simulink library "LateralControl_fcns_lib"  (R2018b)
settings: Solver=ode45  StartTime=0.0  StopTime=10.0  RelTol=1e-3  EnableMultiTasking=on
values from neighbouring files (symbols this model uses):
  c_BIT0 = 1.0    [LCK_LogicPara.sldd]
  c_BIT1 = 2.0    [LCK_LogicPara.sldd]
  c_BIT10 = 1024.0    [LCK_LogicPara.sldd]
  c_BIT11 = 2048.0    [LCK_LogicPara.sldd]
  c_BIT12 = 4096.0    [LCK_LogicPara.sldd]
  c_BIT13 = 8192.0    [LCK_LogicPara.sldd]
  c_BIT14 = 16384.0    [LCK_LogicPara.sldd]
  c_BIT15 = 32768.0    [LCK_LogicPara.sldd]
  c_BIT2 = 4.0    [LCK_LogicPara.sldd]
  c_BIT3 = 8.0    [LCK_LogicPara.sldd]
  c_BIT4 = 16.0    [LCK_LogicPara.sldd]
  c_BIT5 = 32.0    [LCK_LogicPara.sldd]
  c_BIT6 = 64.0    [LCK_LogicPara.sldd]
  c_BIT7 = 128.0    [LCK_LogicPara.sldd]
  c_BIT8 = 256.0    [LCK_LogicPara.sldd]
  c_BIT9 = 512.0    [LCK_LogicPara.sldd]
  ML_TIME_MSEC = 20.0    [LCK_Macro.sldd]
undefined symbols (not defined in the file or in its folder): k_LCK_Valid_Range_Remain_Tm_s, k_SPP_clearance_FusGdr, k_SPP_clearance_RE, k_SPP_clearance_VisBarr, TJA_SP_CONF_LOW
libraries: $bdroot x4, simulink x3, tllib x1
(part 1 of 2)
settings Model: TLRevision=101  Creator=kz0hq6  LastModifiedBy=chenx
settings DataIOCC: LimitDataPoints=on  SaveFormat=Array  SignalLoggingSaveFormat=ModelDataLogs
settings OptimizationCC: ExpressionDepthLimit=2147483647  LifeSpan=inf
settings DebuggingCC: UnderspecifiedInitializationDetection=Classic  MergeDetectMultiDrivingBlocksExec=none  SolverPrmCheckMsg=warning  FcnCallInpInsideContextMsg=warning  AllowSymbolicDim=off  StateNameClashWarn=warning  SFUnexpectedBacktrackingDiag=warning  SFNoUnconditionalDefaultTransitionDiag=warning  SFExecutionAtInitializationDiag=none
settings HardwareCC: ProdBitPerPointer=32  ProdBitPerSizeT=32  ProdBitPerPtrDiffT=32  ProdLargestAtomicFloat=None  ProdIntDivRoundTo=Undefined  ProdEndianess=Unspecified  ProdWordSize=32  ProdHWDeviceType=32-bit Generic
settings ModelReferenceCC: PropagateSignalLabelsOutOfModel=off
settings SFSimCC: SimUseLocalCustomCode=off
settings RTWCC: RTWUseLocalCustomCode=off
settings CodeAppCC: StateflowObjectComments=on
settings GRTTargetCC: TargetLangStandard=C89/C90 (ANSI)  GeneratePreprocessorConditionals=Disable all
settings ConfigComp: CovMetricSettings=dw  CovHtmlReporting=on  CovSaveCumulativeToWorkspaceVar=on  CovSaveSingleToWorkspaceVar=on  CovExternalEMLEnable=off

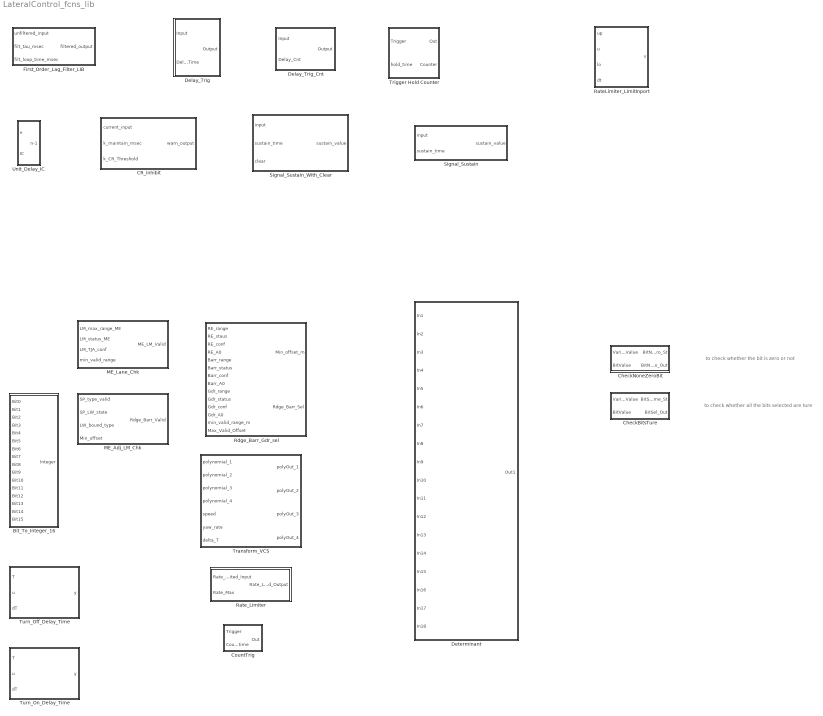
== system LateralControl_fcns_lib ==
  note: to check whether all the bits selected are ture
  note: to check whether the bit is zero or not
  Bit_To_Integer_16 : Subsystem
  CR_inhibit : Subsystem  Description=_GWMAB30P4.Latctrl.000_128_
  CheckBitsTure : Subsystem
  CheckNoneZeroBit : Subsystem
  CountTrig : Subsystem
  Delay_Trig : Subsystem
  Delay_Trig_Cnt : Subsystem  Description=_GWMAB30P4.LKAFN.000_28_
  Determinant : Subsystem
  First_Order_Lag_Filter_LIB : Subsystem
  ME_Adj_LM_Chk : Subsystem
  ME_Lane_Chk : Subsystem
  RateLimiter_LimitInport : Subsystem  mask(Rate Limiter){}
      mask help: Limit rising and falling rates of the signals at the second input by using the first input (upper limit) and the fourth input (lower limit).
      settings: AttributesFormatString=<Rate Limiter>
      mask Display: plot([0.15 0.95],[.5 .5],[.5 .5],[0.05 0.95],0.05+0.9*[.2 .8],0.05+0.9*[0 1]);
  Rate_Limiter : Subsystem  TreatAsAtomicUnit=on
  Rdge_Barr_Gdr_sel : Subsystem
  Signal_Sustain : Subsystem  Description=_GWMAB30P4.LKAFN.000_315_
  Signal_Sustain_With_Clear : Subsystem  Description=_GWMAB30P4.Latctrl.000_162_
  Transform_VCS : Subsystem
  Trigger Hold Counter : Subsystem
  Turn_Off_Delay_Time : Subsystem  mask(TurnOffDelayTime){}
      mask help:
      | The falling edge of the input signal (u) is delayed by the input delay time (T).
      | Input1= Delay Time;  Input2=Signal (u);  Input3=Activation Rate.
      settings: RTWSystemCode=Inline
      mask Help: web(char(which([char(get_param(gcb,'MaskType')),'.html'])));
      mask Display:
      | plot([0.15 0.5 0.5 0.85],[0.9 0.9 0.1 0.1])
      | plot([0.2 0.45],[0.65 0.65])
      | plot([0.325 0.325],[0.65 0.2])
      | port_label('input',1,'T')
      | port_label('input',2,'u')
      | port_label('input',3,'dT')
  Turn_On_Delay_Time : Subsystem  mask(TurnOnDelayTime){}
      mask help: The rising edge of the input signal (u) is delayed by the input delay time (T). Input1= Delay Time; Input2=Signal (u); Input3=Activation Rate.
      settings: RTWSystemCode=Inline
      mask Help: web(char(which([char(get_param(gcb,'MaskType')),'.html'])));
      mask Display:
      | plot([0.15 0.5 0.5 0.85],[0.1 0.1 0.9 0.9])
      | plot([0.55 0.8],[0.65 0.65])
      | plot([0.675 0.675],[0.65 0.2])
      | port_label('input',1,'T')
      | port_label('input',2,'u')
      | port_label('input',3,'dT')
  Unit_Delay_IC : Subsystem

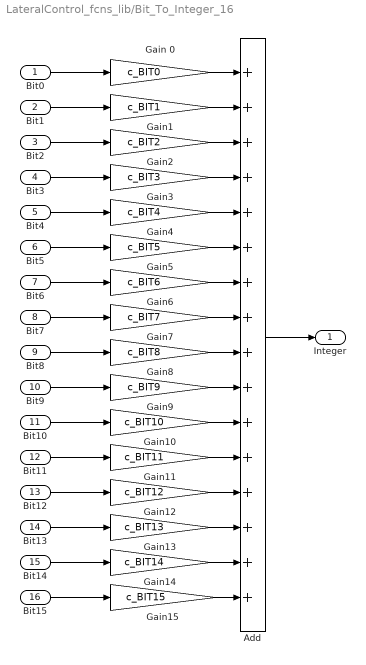
== system LateralControl_fcns_lib/Bit_To_Integer_16 ==
  Bit0 : Inport  Description=_GWMH9P3.LCKFN.000_1_
  Bit1 : Inport  Description=_GWMH9P3.LCKFN.000_2_  Port=2
  Bit2 : Inport  Description=_GWMH9P3.LCKFN.000_3_  Port=3
  Bit3 : Inport  Description=_GWMH9P3.LCKFN.000_4_  Port=4
  Bit4 : Inport  Description=_GWMH9P3.LCKFN.000_5_  Port=5
  Bit5 : Inport  Description=_GWMH9P3.LCKFN.000_6_  Port=6
  Bit6 : Inport  Description=_GWMH9P3.LCKFN.000_7_  Port=7
  Bit7 : Inport  Description=_GWMH9P3.LCKFN.000_8_  Port=8
  Bit8 : Inport  Description=_GWMH9P3.LCKFN.000_9_  Port=9
  Bit9 : Inport  Description=_GWMH9P3.LCKFN.000_10_  Port=10
  Bit10 : Inport  Description=_GWMH9P3.LCKFN.000_11_  Port=11
  Bit11 : Inport  Description=_GWMH9P3.LCKFN.000_12_  Port=12
  Bit12 : Inport  Description=_GWMH9P3.LCKFN.000_13_  Port=13
  Bit13 : Inport  Description=_GWMH9P3.LCKFN.000_14_  Port=14
  Bit14 : Inport  Description=_GWMH9P3.LCKFN.000_15_  Port=15
  Bit15 : Inport  Description=_GWMH9P3.LCKFN.000_16_  Port=16
  Add : Sum  Tag={'output',{'type','UInt16'},'date',737243.50070405088}  Description=_GWMAB30P3.LCKFN.000_1_  Inputs=++++++++++++++++  AccumDataTypeStr=uint16  OutDataTypeStr=uint16
  Gain 0 : Gain  Tag={'output',{'type','UInt16'},'gain',{'name','$P','class','EXTERN_CONST','type','UInt16'},'date',737243.62802085653}  Description=_GWMAB30P3.LCKFN.000_2_  Gain=c_BIT0  ParamDataTypeStr=uint16  OutDataTypeStr=uint16
  Gain1 : Gain  Tag={'output',{'type','UInt16'},'gain',{'name','$P','class','EXTERN_CONST','type','UInt16'},'date',737243.62814724538}  Description=_GWMAB30P3.LCKFN.000_3_  Gain=c_BIT1  ParamDataTypeStr=uint16  OutDataTypeStr=uint16
  Gain10 : Gain  Tag={'output',{'type','UInt16'},'gain',{'name','$P','class','EXTERN_CONST','type','UInt16'},'date',737243.63142819447}  Description=_GWMAB30P3.LCKFN.000_4_  Gain=c_BIT10  ParamDataTypeStr=uint16  OutDataTypeStr=uint16
  Gain11 : Gain  Tag={'output',{'type','UInt16'},'gain',{'name','$P','class','EXTERN_CONST','type','UInt16'},'date',737243.63154284726}  Description=_GWMAB30P3.LCKFN.000_5_  Gain=c_BIT11  ParamDataTypeStr=uint16  OutDataTypeStr=uint16
  Gain12 : Gain  Tag={'output',{'type','UInt16'},'gain',{'name','$P','class','EXTERN_CONST','type','UInt16'},'date',737243.63166906254}  Description=_GWMAB30P3.LCKFN.000_6_  Gain=c_BIT12  ParamDataTypeStr=uint16  OutDataTypeStr=uint16
  Gain13 : Gain  Tag={'output',{'type','UInt16'},'gain',{'name','$P','class','EXTERN_CONST','type','UInt16'},'date',737243.63180953707}  Description=_GWMAB30P3.LCKFN.000_7_  Gain=c_BIT13  ParamDataTypeStr=uint16  OutDataTypeStr=uint16
  Gain14 : Gain  Tag={'output',{'type','UInt16'},'gain',{'name','$P','class','EXTERN_CONST','type','UInt16'},'date',737243.63191913196}  Description=_GWMAB30P3.LCKFN.000_8_  Gain=c_BIT14  ParamDataTypeStr=uint16  OutDataTypeStr=uint16
  Gain15 : Gain  Tag={'output',{'type','UInt16'},'gain',{'name','$P','class','EXTERN_CONST','type','UInt16'},'date',737243.63202458329}  Description=_GWMAB30P3.LCKFN.000_9_  Gain=c_BIT15  ParamDataTypeStr=uint16  OutDataTypeStr=uint16
  Gain2 : Gain  Tag={'output',{'type','UInt16'},'gain',{'name','$P','class','EXTERN_CONST','type','UInt16'},'date',737243.62828194443}  Description=_GWMAB30P3.LCKFN.000_10_  Gain=c_BIT2  ParamDataTypeStr=uint16  OutDataTypeStr=uint16
  Gain3 : Gain  Tag={'output',{'type','UInt16'},'gain',{'name','$P','class','EXTERN_CONST','type','UInt16'},'date',737243.62842260418}  Description=_GWMAB30P3.LCKFN.000_11_  Gain=c_BIT3  ParamDataTypeStr=uint16  OutDataTypeStr=uint16
  Gain4 : Gain  Tag={'output',{'type','UInt16'},'gain',{'name','$P','class','EXTERN_CONST','type','UInt16'},'date',737243.63042121532}  Description=_GWMAB30P3.LCKFN.000_12_  Gain=c_BIT4  ParamDataTypeStr=uint16  OutDataTypeStr=uint16
  Gain5 : Gain  Tag={'output',{'type','UInt16'},'gain',{'name','$P','class','EXTERN_CONST','type','UInt16'},'date',737243.63074442127}  Description=_GWMAB30P3.LCKFN.000_13_  Gain=c_BIT5  ParamDataTypeStr=uint16  OutDataTypeStr=uint16
  Gain6 : Gain  Tag={'output',{'type','UInt16'},'gain',{'name','$P','class','EXTERN_CONST','type','UInt16'},'date',737243.63092443289}  Description=_GWMAB30P3.LCKFN.000_14_  Gain=c_BIT6  ParamDataTypeStr=uint16  OutDataTypeStr=uint16
  Gain7 : Gain  Tag={'output',{'type','UInt16'},'gain',{'name','$P','class','EXTERN_CONST','type','UInt16'},'date',737243.63104162039}  Description=_GWMAB30P3.LCKFN.000_15_  Gain=c_BIT7  ParamDataTypeStr=uint16  OutDataTypeStr=uint16
  Gain8 : Gain  Tag={'output',{'type','UInt16'},'gain',{'name','$P','class','EXTERN_CONST','type','UInt16'},'date',737243.63116565975}  Description=_GWMAB30P3.LCKFN.000_16_  Gain=c_BIT8  ParamDataTypeStr=uint16  OutDataTypeStr=uint16
  Gain9 : Gain  Tag={'output',{'type','UInt16'},'gain',{'name','$P','class','EXTERN_CONST','type','UInt16'},'date',737243.63129422453}  Description=_GWMAB30P3.LCKFN.000_17_  Gain=c_BIT9  ParamDataTypeStr=uint16  OutDataTypeStr=uint16
  Integer : Outport  Description=_GWMH9P3.LCKFN.000_17_
  wires:
  Gain 0/1 -> Add/1
  Gain1/1 -> Add/2
  Gain2/1 -> Add/3
  Gain3/1 -> Add/4
  Gain4/1 -> Add/5
  Gain5/1 -> Add/6
  Gain6/1 -> Add/7
  Gain7/1 -> Add/8
  Gain8/1 -> Add/9
  Gain9/1 -> Add/10
  Gain10/1 -> Add/11
  Gain11/1 -> Add/12
  Gain12/1 -> Add/13
  Gain13/1 -> Add/14
  Gain14/1 -> Add/15
  Gain15/1 -> Add/16
  Add/1 -> Integer/1
  Bit0/1 -> Gain 0/1
  Bit1/1 -> Gain1/1
  Bit2/1 -> Gain2/1
  Bit3/1 -> Gain3/1
  Bit4/1 -> Gain4/1
  Bit5/1 -> Gain5/1
  Bit6/1 -> Gain6/1
  Bit7/1 -> Gain7/1
  Bit8/1 -> Gain8/1
  Bit9/1 -> Gain9/1
  Bit10/1 -> Gain10/1
  Bit11/1 -> Gain11/1
  Bit12/1 -> Gain12/1
  Bit13/1 -> Gain13/1
  Bit14/1 -> Gain14/1
  Bit15/1 -> Gain15/1

== system LateralControl_fcns_lib/CR_inhibit ==
  current_input : Inport  Description=_GWMAB30P4.LKAFN.000_2_
  k_maintain_msec : Inport  Description=_GWMAB30P4.LKAFN.000_3_  Port=2
  k_CR_Threshold : Inport  Description=_GWMAB30P4.LKAFN.000_4_  Port=3
  CR_inhibit : Stateflow chart  Description=_GWMAB30P4.LKAFN.000_5_  TreatAsAtomicUnit=on
  warn_output : Outport  Description=_GWMAB30P4.LKAFN.000_10_
  wires:
  k_CR_Threshold/1 -> CR_inhibit/3(k_CR_Threshold)
  k_maintain_msec/1 -> CR_inhibit/2(k_mantian_msec)
  current_input/1 -> CR_inhibit/1(current_input)
  CR_inhibit/1(warn_output) -> warn_output/1

== system LateralControl_fcns_lib/CheckBitsTure ==
  VariableValue : Inport
  BitValue : Inport  Port=2
  Bitwise Operator5 : simulink/Logic and Bit Operations/Bitwise Operator  logicop=AND  UseBitMask=off  NumInputPorts=2  BitMask=bin2dec('11011001')  BitMaskRealWorld=Stored Integer
  Data Type Conversion26 : DataTypeConversion
  Relational_Operator4 : RelationalOperator  Operator===  OutDataTypeStr=boolean  RndMeth=Nearest
  BitSelSame_St : Outport
  BitSel_Out : Outport  Port=2
  wires:
  BitValue/1 -> Relational_Operator4/2, Data Type Conversion26/1
  VariableValue/1 -> Bitwise Operator5/1
  Relational_Operator4/1 -> BitSelSame_St/1
  Data Type Conversion26/1 -> Bitwise Operator5/2
  Bitwise Operator5/1 -> BitSel_Out/1, Relational_Operator4/1

== system LateralControl_fcns_lib/CheckNoneZeroBit ==
  VariableValue : Inport
  BitValue : Inport  Port=2
  Bitwise AND : simulink/Logic and Bit Operations/Bitwise Operator  logicop=AND  UseBitMask=off  NumInputPorts=2  BitMask=bin2dec('11011001')  BitMaskRealWorld=Stored Integer
  Constant8 : Constant  Value=0
  Data Type Conversion : DataTypeConversion
  Data Type Conversion2 : DataTypeConversion  OutDataTypeStr=uint16
  Relational Operator14 : RelationalOperator  Operator=~=  OutDataTypeStr=boolean  RndMeth=Nearest
  BitNZero_St : Outport
  BitNZero_Out : Outport  Port=2
  wires:
  Data Type Conversion/1 -> Bitwise AND/2
  Relational Operator14/1 -> BitNZero_St/1
  Constant8/1 -> Relational Operator14/2
  BitValue/1 -> Data Type Conversion/1
  Bitwise AND/1 -> Data Type Conversion2/1, Relational Operator14/1
  Data Type Conversion2/1 -> BitNZero_Out/1
  VariableValue/1 -> Bitwise AND/1

== system LateralControl_fcns_lib/CountTrig ==
  Trigger : Inport  Description=_GWMH9P4.LCKFN.000_1_
  Counttrig_time : Inport  Description=_GWMH9P4.LCKFN.000_2_  Port=2
  CountTrig : Stateflow chart  TreatAsAtomicUnit=on
  Out : Outport  Description=_GWMH9P4.LCKFN.000_6_
  wires:
  CountTrig/1(Out) -> Out/1
  Counttrig_time/1 -> CountTrig/2(CountTrig_time)
  Trigger/1 -> CountTrig/1(Trigger)

== system LateralControl_fcns_lib/Delay_Trig ==
  Input : Inport  Description=_GWMH9P3.LCKFN.000_18_
  Delay_Trig_Time : Inport  Description=_GWMH9P3.LCKFN.000_19_  Port=2
  Delay_Trig : Stateflow chart  TreatAsAtomicUnit=on
  Output : Outport  Description=_GWMH9P3.LCKFN.000_23_
  wires:
  Input/1 -> Delay_Trig/1(Input)
  Delay_Trig_Time/1 -> Delay_Trig/2(Delay_Trig_Time)
  Delay_Trig/1(Delay_Trig) -> Output/1

== system LateralControl_fcns_lib/Delay_Trig_Cnt ==
  Input : Inport  Description=_GWMAB30P4.LKAFN.000_29_
  Delay_Cnt : Inport  Description=_GWMAB30P4.LKAFN.000_30_  Port=2
  Delay_Trig : Stateflow chart  Description=_GWMAB30P4.LKAFN.000_31_  TreatAsAtomicUnit=on
  Output : Outport  Description=_GWMAB30P4.LKAFN.000_35_
  wires:
  Delay_Cnt/1 -> Delay_Trig/2(Delay_Trig_count)
  Delay_Trig/1(Delay_Trig) -> Output/1
  Input/1 -> Delay_Trig/1(Input)

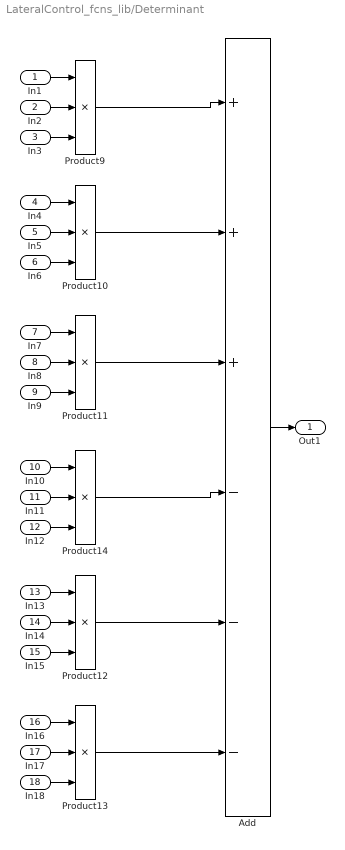
== system LateralControl_fcns_lib/Determinant ==
  In1 : Inport  Tag={'output',{'type','Float32'},'date',737464.8958215625}  Description=_GWMH9P4.LCKFN.000_10_
  In2 : Inport  Tag={'output',{'type','Float32'},'date',737464.8958774074}  Description=_GWMH9P4.LCKFN.000_11_  Port=2
  In3 : Inport  Tag={'output',{'type','Float32'},'date',737464.89607775467}  Description=_GWMH9P4.LCKFN.000_12_  Port=3
  In4 : Inport  Tag={'output',{'type','Float32'},'date',737464.8961349884}  Description=_GWMH9P4.LCKFN.000_13_  Port=4
  In5 : Inport  Tag={'output',{'type','Float32'},'date',737464.89620260417}  Description=_GWMH9P4.LCKFN.000_14_  Port=5
  In6 : Inport  Tag={'output',{'type','Float32'},'date',737464.89625967597}  Description=_GWMH9P4.LCKFN.000_15_  Port=6
  In7 : Inport  Tag={'output',{'type','Float32'},'date',737464.89632886578}  Description=_GWMH9P4.LCKFN.000_16_  Port=7
  In8 : Inport  Tag={'output',{'type','Float32'},'date',737464.89639204857}  Description=_GWMH9P4.LCKFN.000_17_  Port=8
  In9 : Inport  Tag={'output',{'type','Float32'},'date',737464.89645353006}  Description=_GWMH9P4.LCKFN.000_18_  Port=9
  In10 : Inport  Tag={'output',{'type','Float32'},'date',737464.89651208336}  Description=_GWMH9P4.LCKFN.000_19_  Port=10
  In11 : Inport  Tag={'output',{'type','Float32'},'date',737464.89657822915}  Description=_GWMH9P4.LCKFN.000_20_  Port=11
  In12 : Inport  Tag={'output',{'type','Float32'},'date',737464.8966244444}  Description=_GWMH9P4.LCKFN.000_21_  Port=12
  In13 : Inport  Tag={'output',{'type','Float32'},'date',737464.896679456}  Description=_GWMH9P4.LCKFN.000_22_  Port=13
  In14 : Inport  Tag={'output',{'type','Float32'},'date',737464.89673541661}  Description=_GWMH9P4.LCKFN.000_23_  Port=14
  In15 : Inport  Tag={'output',{'type','Float32'},'date',737464.89679289353}  Description=_GWMH9P4.LCKFN.000_24_  Port=15
  In16 : Inport  Tag={'output',{'type','Float32'},'date',737464.89685541671}  Description=_GWMH9P4.LCKFN.000_25_  Port=16
  In17 : Inport  Tag={'output',{'type','Float32'},'date',737464.89690805553}  Description=_GWMH9P4.LCKFN.000_26_  Port=17
  In18 : Inport  Tag={'output',{'type','Float32'},'date',737464.89696628472}  Description=_GWMH9P4.LCKFN.000_27_  Port=18
  Add : Sum  Tag={'output',{'type','Float32'},'date',737462.84083193284}  Description=_GWMH9P4.LCKFN.000_28_  Inputs=+++---
  Product10 : Product  Tag={'output',{'type','Float32'},'date',737462.84057671297}  Description=_GWMH9P4.LCKFN.000_29_  Inputs=3  RndMeth=Zero
  Product11 : Product  Tag={'output',{'type','Float32'},'date',737462.8406229167}  Description=_GWMH9P4.LCKFN.000_30_  Inputs=3  RndMeth=Zero
  Product12 : Product  Tag={'output',{'type','Float32'},'date',737462.84072949074}  Description=_GWMH9P4.LCKFN.000_31_  Inputs=3  RndMeth=Zero
  Product13 : Product  Tag={'output',{'type','Float32'},'date',737462.84078811342}  Description=_GWMH9P4.LCKFN.000_32_  Inputs=3  RndMeth=Zero
  Product14 : Product  Tag={'output',{'type','Float32'},'date',737462.84066295135}  Description=_GWMH9P4.LCKFN.000_33_  Inputs=3  RndMeth=Zero
  Product9 : Product  Tag={'output',{'type','Float32'},'date',737462.8405174769}  Description=_GWMH9P4.LCKFN.000_34_  Inputs=3  RndMeth=Zero
  Out1 : Outport  Tag={'output',{'name','Determinant_out','class','ESR_VC/FCN_RETURN','type','Float32'},'date',737464.89569219912}  Description=_GWMH9P4.LCKFN.000_35_
  wires:
  Product9/1 -> Add/1
  Product10/1 -> Add/2
  Product11/1 -> Add/3
  Product14/1 -> Add/4
  Product12/1 -> Add/5
  Product13/1 -> Add/6
  In1/1 -> Product9/1
  In2/1 -> Product9/2
  In3/1 -> Product9/3
  In4/1 -> Product10/1
  In5/1 -> Product10/2
  In6/1 -> Product10/3
  In7/1 -> Product11/1
  In8/1 -> Product11/2
  In9/1 -> Product11/3
  Add/1 -> Out1/1
  In10/1 -> Product14/1
  In11/1 -> Product14/2
  In12/1 -> Product14/3
  In13/1 -> Product12/1
  In14/1 -> Product12/2
  In15/1 -> Product12/3
  In16/1 -> Product13/1
  In17/1 -> Product13/2
  In18/1 -> Product13/3

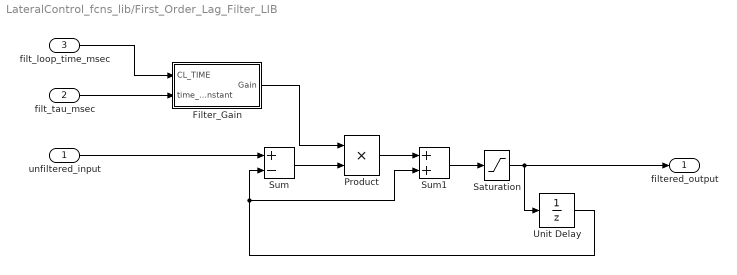
== system LateralControl_fcns_lib/First_Order_Lag_Filter_LIB ==
  unfiltered_input : Inport  Description=_GWMAB30P4.LKAFN.000_148_
  filt_tau_msec : Inport  Description=_GWMAB30P4.LKAFN.000_149_  Port=2
  filt_loop_time_msec : Inport  Description=_GWMAB30P4.LKAFN.000_150_  Port=3
  Filter_Gain : Subsystem
  Product : Product  Description=_GWMAB30P4.LKAFN.000_153_  Inputs=**
  Saturation : Saturate  Description=_GWMAB30P4.LKAFN.000_154_  UpperLimit=65535  LowerLimit=-65535
  Sum : Sum  Description=_GWMAB30P4.LKAFN.000_155_  Inputs=+-  OutDataTypeStr=Inherit: Same as first input
  Sum1 : Sum  Description=_GWMAB30P4.LKAFN.000_156_  OutDataTypeStr=Inherit: Same as first input
  Unit Delay : UnitDelay  Description=_GWMAB30P4.LKAFN.000_157_  SampleTime=-1
  filtered_output : Outport  Description=_GWMAB30P4.LKAFN.000_158_
  wires:
  Filter_Gain/1(Gain) -> Product/1
  Saturation/1 -> filtered_output/1, Unit Delay/1
  Unit Delay/1 -> Sum1/2, Sum/2
  Sum/1 -> Product/2
  Sum1/1 -> Saturation/1
  unfiltered_input/1 -> Sum/1
  filt_tau_msec/1 -> Filter_Gain/2(time_constant)
  Product/1 -> Sum1/1
  filt_loop_time_msec/1 -> Filter_Gain/1(CL_TIME)

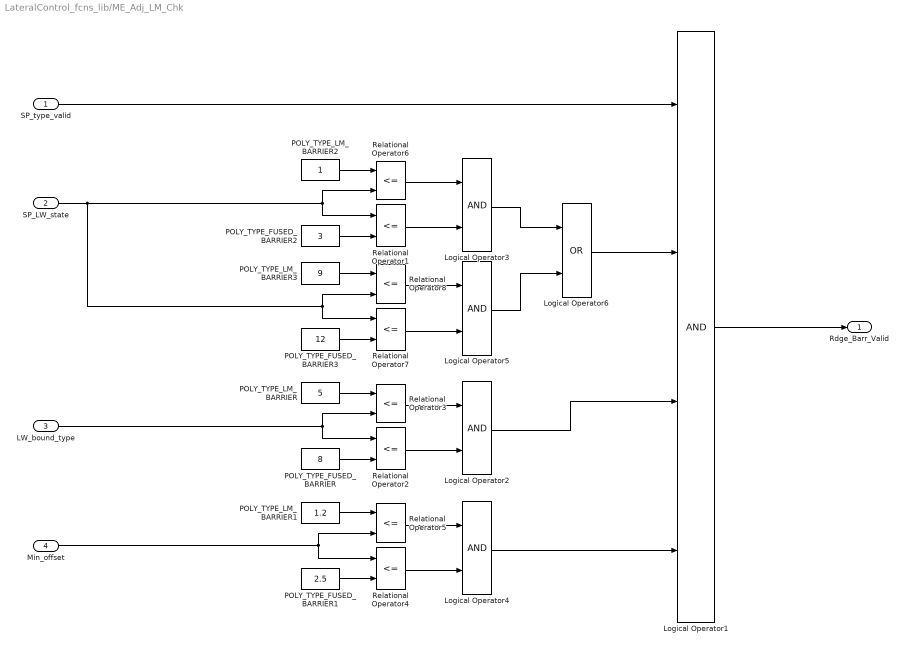
== system LateralControl_fcns_lib/ME_Adj_LM_Chk ==
  SP_type_valid : Inport  Description=_GWMH9P3.LCKFN.000_24_
  SP_LW_state : Inport  Description=_GWMH9P3.LCKFN.000_25_  Port=2
  LW_bound_type : Inport  Description=_GWMH9P3.LCKFN.000_26_  Port=3
  Min_offset : Inport  Description=_GWMH9P3.LCKFN.000_27_  Port=4
  Logical Operator1 : Logic  Tag={'date',737393.51890250004}  Description=_GWMH9P3.LCKFN.000_28_  Inputs=4  AllPortsSameDT=off  OutDataTypeStr=boolean
  Logical Operator2 : Logic  Tag={'date',737393.51890320599}  Description=_GWMH9P3.LCKFN.000_29_  AllPortsSameDT=off  OutDataTypeStr=boolean
  Logical Operator3 : Logic  Tag={'date',737393.51890342589}  Description=_GWMH9P3.LCKFN.000_30_  AllPortsSameDT=off  OutDataTypeStr=boolean
  Logical Operator4 : Logic  Tag={'date',737393.5189036458}  Description=_GWMH9P3.LCKFN.000_31_  AllPortsSameDT=off  OutDataTypeStr=boolean
  Logical Operator5 : Logic  Tag={'date',737393.51890388888}  Description=_GWMH9P3.LCKFN.000_32_  AllPortsSameDT=off  OutDataTypeStr=boolean
  Logical Operator6 : Logic  Tag={'date',737393.51890412043}  Description=_GWMH9P3.LCKFN.000_33_  Operator=OR  AllPortsSameDT=off  OutDataTypeStr=boolean
  POLY_TYPE_FUSED_BARRIER : Constant  Tag={'output',{'type','Int32'},'date',737393.51890491904}  Description=_GWMH9P3.LCKFN.000_34_  Value=8  SampleTime=-1
  POLY_TYPE_FUSED_BARRIER1 : Constant  Tag={'output',{'type','Int32'},'date',737393.51890531252}  Description=_GWMH9P3.LCKFN.000_35_  Value=2.5  SampleTime=-1
  POLY_TYPE_FUSED_BARRIER2 : Constant  Tag={'output',{'type','Int32'},'date',737393.5189055556}  Description=_GWMH9P3.LCKFN.000_36_  Value=3  SampleTime=-1
  POLY_TYPE_FUSED_BARRIER3 : Constant  Tag={'output',{'type','Int32'},'date',737393.51890578703}  Description=_GWMH9P3.LCKFN.000_37_  Value=12  SampleTime=-1
  POLY_TYPE_LM_BARRIER : Constant  Tag={'output',{'type','Int32'},'date',737393.51890601846}  Description=_GWMH9P3.LCKFN.000_38_  Value=5  SampleTime=-1
  POLY_TYPE_LM_BARRIER1 : Constant  Tag={'output',{'type','Int32'},'date',737393.51890626154}  Description=_GWMH9P3.LCKFN.000_39_  Value=1.2  SampleTime=-1
  POLY_TYPE_LM_BARRIER2 : Constant  Tag={'output',{'type','Int32'},'date',737393.51890650461}  Description=_GWMH9P3.LCKFN.000_40_  SampleTime=-1
  POLY_TYPE_LM_BARRIER3 : Constant  Tag={'output',{'type','Int32'},'date',737393.51890672452}  Description=_GWMH9P3.LCKFN.000_41_  Value=9  SampleTime=-1
  Relational Operator1 : RelationalOperator  Tag={'date',737393.51890695607}  Description=_GWMH9P3.LCKFN.000_42_  Operator=<=  OutDataTypeStr=boolean  RndMeth=Nearest
  Relational Operator2 : RelationalOperator  Tag={'date',737393.51890716434}  Description=_GWMH9P3.LCKFN.000_43_  Operator=<=  OutDataTypeStr=boolean  RndMeth=Nearest
  Relational Operator3 : RelationalOperator  Tag={'date',737393.51890737272}  Description=_GWMH9P3.LCKFN.000_44_  Operator=<=  OutDataTypeStr=boolean  RndMeth=Nearest
  Relational Operator4 : RelationalOperator  Tag={'date',737393.51890755782}  Description=_GWMH9P3.LCKFN.000_45_  Operator=<=  OutDataTypeStr=boolean  RndMeth=Nearest
  Relational Operator5 : RelationalOperator  Tag={'date',737393.51890776621}  Description=_GWMH9P3.LCKFN.000_46_  Operator=<=  OutDataTypeStr=boolean  RndMeth=Nearest
  Relational Operator6 : RelationalOperator  Tag={'date',737393.51890796295}  Description=_GWMH9P3.LCKFN.000_47_  Operator=<=  OutDataTypeStr=boolean  RndMeth=Nearest
  Relational Operator7 : RelationalOperator  Tag={'date',737393.51890815969}  Description=_GWMH9P3.LCKFN.000_48_  Operator=<=  OutDataTypeStr=boolean  RndMeth=Nearest
  Relational Operator8 : RelationalOperator  Tag={'date',737393.51890836807}  Description=_GWMH9P3.LCKFN.000_49_  Operator=<=  OutDataTypeStr=boolean  RndMeth=Nearest
  Rdge_Barr_Valid : Outport  Description=_GWMH9P3.LCKFN.000_50_
  wires:
  Logical Operator1/1 -> Rdge_Barr_Valid/1
  LW_bound_type/1 -> Relational Operator2/1, Relational Operator3/2
  POLY_TYPE_FUSED_BARRIER/1 -> Relational Operator2/2
  POLY_TYPE_LM_BARRIER/1 -> Relational Operator3/1
  Relational Operator2/1 -> Logical Operator2/2
  Relational Operator3/1 -> Logical Operator2/1
  Min_offset/1 -> Relational Operator5/2, Relational Operator4/1
  POLY_TYPE_FUSED_BARRIER1/1 -> Relational Operator4/2
  POLY_TYPE_LM_BARRIER1/1 -> Relational Operator5/1
  Relational Operator4/1 -> Logical Operator4/2
  Relational Operator5/1 -> Logical Operator4/1
  SP_LW_state/1 -> Relational Operator6/2, Relational Operator1/1, Relational Operator7/1, Relational Operator8/2
  POLY_TYPE_FUSED_BARRIER2/1 -> Relational Operator1/2
  POLY_TYPE_LM_BARRIER2/1 -> Relational Operator6/1
  Relational Operator1/1 -> Logical Operator3/2
  Relational Operator6/1 -> Logical Operator3/1
  POLY_TYPE_FUSED_BARRIER3/1 -> Relational Operator7/2
  POLY_TYPE_LM_BARRIER3/1 -> Relational Operator8/1
  Relational Operator7/1 -> Logical Operator5/2
  Relational Operator8/1 -> Logical Operator5/1
  Logical Operator3/1 -> Logical Operator6/1
  Logical Operator5/1 -> Logical Operator6/2
  SP_type_valid/1 -> Logical Operator1/1
  Logical Operator6/1 -> Logical Operator1/2
  Logical Operator2/1 -> Logical Operator1/3
  Logical Operator4/1 -> Logical Operator1/4

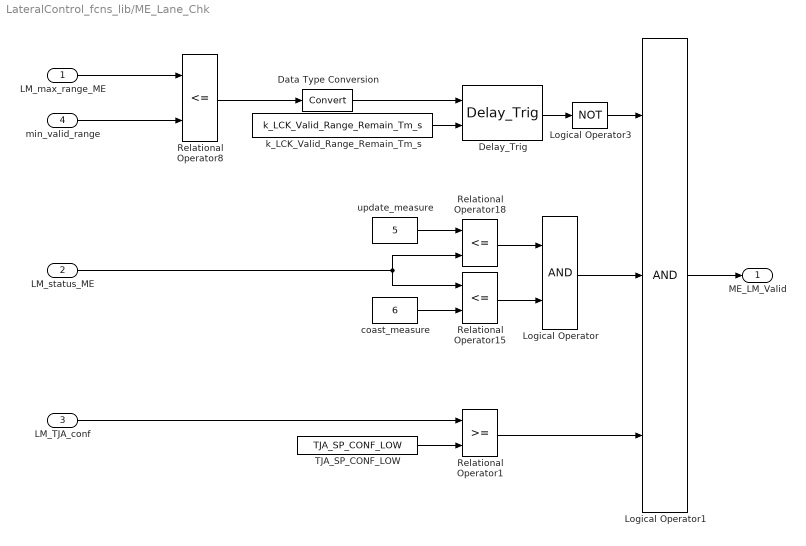
== system LateralControl_fcns_lib/ME_Lane_Chk ==
  LM_max_range_ME : Inport  Tag={'output',{'name','$I_LM_max_range_ME','type','Float32'},'date',737429.7295920949}  Description=_GWMH9P3.LCKFN.000_51_
  LM_status_ME : Inport  Tag={'output',{'name','$I_LM_status_ME','type','UInt8'},'date',737429.72993736109}  Description=_GWMH9P3.LCKFN.000_52_  Port=2
  LM_TJA_conf : Inport  Tag={'output',{'name','$I_LM_TJA_conf','type','UInt8'},'date',737429.73083754629}  Description=_GWMH9P3.LCKFN.000_53_  Port=3
  min_valid_range : Inport  Tag={'output',{'name','$I_min_valid_range','type','UInt8'},'date',737429.72976344905}  Description=_GWMH9P3.LCKFN.000_54_  Port=4
  Data Type Conversion : DataTypeConversion  Description=_GWMH9P3.LCKFN.000_55_
  Delay_Trig : $bdroot/Delay_Trig  SystemSampleTime=-1
  Logical Operator : Logic  Tag={'date',737237.63446607639}  Description=_GWMAB30P3.LCKFN.000_18_  AllPortsSameDT=off  OutDataTypeStr=boolean
  Logical Operator1 : Logic  Tag={'date',737237.63446620374}  Description=_GWMAB30P3.LCKFN.000_19_  Inputs=3  AllPortsSameDT=off  OutDataTypeStr=boolean
  Logical Operator3 : Logic  Tag={'date',737237.63446633099}  Description=_GWMAB30P3.LCKFN.000_20_  Operator=NOT  Inputs=1  AllPortsSameDT=off  OutDataTypeStr=boolean
  Relational Operator1 : RelationalOperator  Tag={'date',737237.6344665857}  Description=_GWMAB30P3.LCKFN.000_21_  OutDataTypeStr=boolean  RndMeth=Nearest
  Relational Operator15 : RelationalOperator  Tag={'date',737237.63446671295}  Description=_GWMAB30P3.LCKFN.000_22_  Operator=<=  OutDataTypeStr=boolean  RndMeth=Nearest
  Relational Operator18 : RelationalOperator  Tag={'date',737237.63446682866}  Description=_GWMAB30P3.LCKFN.000_23_  Operator=<=  OutDataTypeStr=boolean  RndMeth=Nearest
  Relational Operator8 : RelationalOperator  Tag={'date',737237.63446693285}  Description=_GWMAB30P3.LCKFN.000_24_  Operator=<=  OutDataTypeStr=boolean  RndMeth=Nearest
  TJA_SP_CONF_LOW : Constant  Tag={'output',{'name','$P','class','EXTERN_MACRO','type','UInt8'},'date',737237.8042558796}  Description=_GWMAB30P3.LCKFN.000_25_  Value=TJA_SP_CONF_LOW  SampleTime=-1
  coast_measure : Constant  Tag={'output',{'type','Int32'},'date',737237.6344671991}  Description=_GWMAB30P3.LCKFN.000_26_  Value=6  SampleTime=-1
  k_LCK_Valid_Range_Remain_Tm_s : Constant  Tag={'output',{'name','$P','class','EXTERN_CAL','type','Float32'},'date',737237.80413560185}  Description=_GWMAB30P3.LCKFN.000_27_  Value=k_LCK_Valid_Range_Remain_Tm_s  SampleTime=-1
  update_measure : Constant  Tag={'output',{'type','Int32'},'date',737237.63446748839}  Description=_GWMAB30P3.LCKFN.000_28_  Value=5  SampleTime=-1
  ME_LM_Valid : Outport  Tag={'output',{'name','$I_ME_LM_Valid','class','ESR_VC/FCN_RETURN','type','Bool'},'date',737429.72934129625}  Description=_GWMH9P3.LCKFN.000_56_
  wires:
  min_valid_range/1 -> Relational Operator8/2
  LM_max_range_ME/1 -> Relational Operator8/1
  LM_status_ME/1 -> Relational Operator18/2, Relational Operator15/1
  coast_measure/1 -> Relational Operator15/2
  update_measure/1 -> Relational Operator18/1
  LM_TJA_conf/1 -> Relational Operator1/1
  TJA_SP_CONF_LOW/1 -> Relational Operator1/2
  Relational Operator15/1 -> Logical Operator/2
  Relational Operator18/1 -> Logical Operator/1
  Logical Operator/1 -> Logical Operator1/2
  Relational Operator1/1 -> Logical Operator1/3
  Logical Operator1/1 -> ME_LM_Valid/1
  Relational Operator8/1 -> Data Type Conversion/1
  Logical Operator3/1 -> Logical Operator1/1
  Delay_Trig/1 -> Logical Operator3/1
  k_LCK_Valid_Range_Remain_Tm_s/1 -> Delay_Trig/2
  Data Type Conversion/1 -> Delay_Trig/1

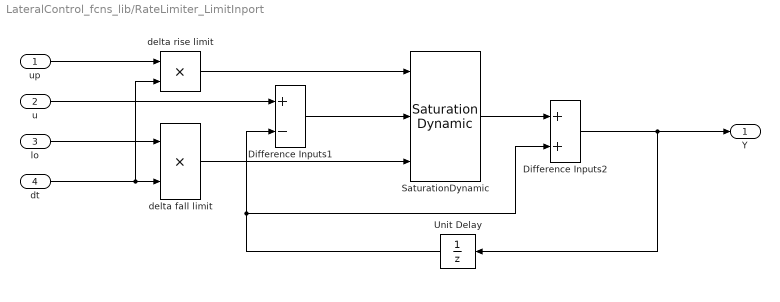
== system LateralControl_fcns_lib/RateLimiter_LimitInport ==
  up : Inport
  u : Inport  Port=2
  lo : Inport  Port=3
  dt : Inport  Port=4
  Difference Inputs1 : Sum  Description=Add in CPU  Inputs=+-  OutDataTypeStr=Inherit: Inherit via back propagation  RndMeth=Zero
  Difference Inputs2 : Sum  Description=Add in CPU  OutDataTypeStr=Inherit: Inherit via back propagation  RndMeth=Zero
  SaturationDynamic : simulink/Discontinuities/Saturation Dynamic  OutMin=[]  OutMax=[]  OutDataTypeStr=Inherit: Same as second input  OutDataType=fixdt(1, 16)  OutScaling=2^-10  RndMeth=Zero  DoSatur=off
  Unit Delay : UnitDelay  SampleTime=-1
  delta fall limit : Product  Inputs=**  OutDataTypeStr=Inherit: Inherit via back propagation  SaturateOnIntegerOverflow=on  RndMeth=Zero
  delta rise limit : Product  Inputs=**  OutDataTypeStr=Inherit: Inherit via back propagation  SaturateOnIntegerOverflow=on  RndMeth=Zero
  Y : Outport  InitialOutput=0
  wires:
  Difference Inputs1/1 -> SaturationDynamic/2
  u/1 -> Difference Inputs1/1
  delta fall limit/1 -> SaturationDynamic/3
  SaturationDynamic/1 -> Difference Inputs2/1
  Unit Delay/1 -> Difference Inputs1/2, Difference Inputs2/2
  Difference Inputs2/1 -> Unit Delay/1, Y/1
  up/1 -> delta rise limit/1
  delta rise limit/1 -> SaturationDynamic/1
  lo/1 -> delta fall limit/1
  dt/1 -> delta fall limit/2, delta rise limit/2

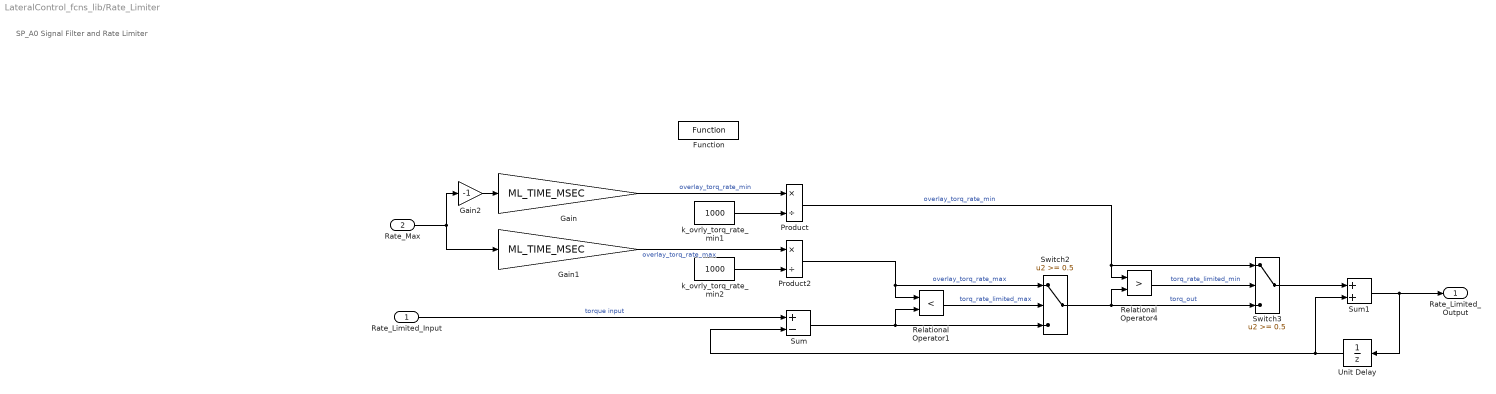
== system LateralControl_fcns_lib/Rate_Limiter ==
  note: SP_A0 Signal Filter and Rate Limiter
  Rate_Limited_Input : Inport  Description=_GWMH9P4.LCKFN.000_36_
  Rate_Max : Inport  Description=_GWMH9P4.LCKFN.000_37_  Port=2
  Function : tllib/Function
  Gain : Gain  Tag={'output',{'type','Float32'},'gain',{'name','$P','class','EXTERN_MACRO','type','ESR_Typedefs/unsigned8_T'},'date',737464.50571820606}  Description=_GWMH9P4.LCKFN.000_38_  Gain=ML_TIME_MSEC
  Gain1 : Gain  Tag={'output',{'type','Float32'},'gain',{'name','$P','class','EXTERN_MACRO','type','ESR_Typedefs/unsigned8_T'},'date',737464.50596844906}  Description=_GWMH9P4.LCKFN.000_39_  Gain=ML_TIME_MSEC
  Gain2 : Gain  Tag={'output',{'type','Float32'},'gain',{'type','Int32'},'date',737462.83431409718}  Description=_GWMH9P4.LCKFN.000_40_  Gain=-1
  Product : Product  Tag={'output',{'type','Float32'},'exceptionhandling',0,'date',737462.83562771988}  Description=_GWMH9P4.LCKFN.000_41_  Inputs=*/  InputSameDT=on  OutDataTypeStr=Inherit: Same as first input
  Product2 : Product  Tag={'output',{'type','Float32'},'exceptionhandling',0,'date',737462.83566040511}  Description=_GWMH9P4.LCKFN.000_42_  Inputs=*/  InputSameDT=on  OutDataTypeStr=Inherit: Same as first input
  Relational Operator1 : RelationalOperator  Tag={'date',737462.49266613426}  Description=_GWMH9P4.LCKFN.000_43_  Operator=<  RndMeth=Nearest
  Relational Operator4 : RelationalOperator  Tag={'date',737462.49266649305}  Description=_GWMH9P4.LCKFN.000_44_  Operator=>  RndMeth=Nearest
  Sum : Sum  Tag={'output',{'type','Float32'},'date',737462.83688239579}  Description=_GWMH9P4.LCKFN.000_45_  Inputs=+-  InputSameDT=on  OutDataTypeStr=Inherit: Same as first input
  Sum1 : Sum  Tag={'output',{'type','Float32'},'date',737462.83708119218}  Description=_GWMH9P4.LCKFN.000_46_  InputSameDT=on  OutDataTypeStr=Inherit: Same as first input
  Switch2 : Switch  Tag={'output',{'type','Float32'},'threshold',{'type','Int32'},'date',737462.8369607986}  Description=_GWMH9P4.LCKFN.000_47_  Threshold=0.5  OutDataTypeStr=Inherit: Inherit via back propagation
  Switch3 : Switch  Tag={'output',{'type','Float32'},'threshold',{'type','Int32'},'date',737462.83703094907}  Description=_GWMH9P4.LCKFN.000_48_  Threshold=0.5  OutDataTypeStr=Inherit: Inherit via back propagation
  Unit Delay : UnitDelay  Tag={'output',{'inheritscaling',1},'date',737462.6251862963}  Description=_GWMH9P4.LCKFN.000_49_  SampleTime=-1
  k_ovrly_torq_rate_min1 : Constant  Tag={'output',{'type','Int32'},'date',737462.8361334838}  Description=_GWMH9P4.LCKFN.000_50_  Value=1000
  k_ovrly_torq_rate_min2 : Constant  Tag={'output',{'type','Int32'},'date',737462.8361574884}  Description=_GWMH9P4.LCKFN.000_51_  Value=1000
  Rate_Limited_Output : Outport  Description=_GWMH9P4.LCKFN.000_52_
  wires:
  k_ovrly_torq_rate_min2/1 -> Product2/2
  Gain1/1 -> Product2/1  "overlay_torq_rate_max"
  k_ovrly_torq_rate_min1/1 -> Product/2
  Gain/1 -> Product/1  "overlay_torq_rate_min"
  Relational Operator1/1 -> Switch2/2  "torq_rate_limited_max"
  Switch2/1 -> Relational Operator4/2, Switch3/3  "torq_out"
  Relational Operator4/1 -> Switch3/2  "torq_rate_limited_min"
  Gain2/1 -> Gain/1
  Product2/1 -> Relational Operator1/1, Switch2/1  "overlay_torq_rate_max"
  Product/1 -> Relational Operator4/1, Switch3/1  "overlay_torq_rate_min"
  Switch3/1 -> Sum1/1
  Sum/1 -> Relational Operator1/2, Switch2/3
  Unit Delay/1 -> Sum/2, Sum1/2
  Sum1/1 -> Rate_Limited_Output/1, Unit Delay/1
  Rate_Limited_Input/1 -> Sum/1  "torque input"
  Rate_Max/1 -> Gain2/1, Gain1/1

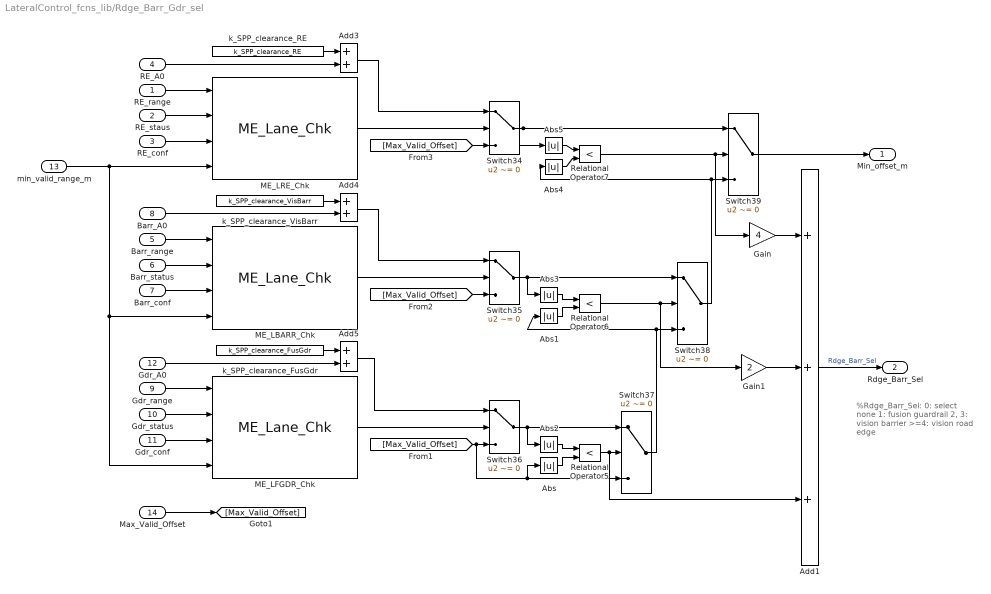
== system LateralControl_fcns_lib/Rdge_Barr_Gdr_sel ==
  note: %Rdge_Barr_Sel:
      | 0:       select none
      | 1:       fusion guardrail
      | 2, 3:   vision barrier
      | >=4:   vision road edge
  RE_range : Inport  Tag={'output',{'name','$I_RE_range','class','ESR_VC/FCN_ARG','type','Float32'},'date',737395.78900525463}  Description=_GWMH9P3.LCKFN.000_57_
  RE_staus : Inport  Tag={'output',{'name','$I_RE_Status','class','ESR_VC/FCN_ARG','type','UInt8'},'date',737395.7890536458}  Description=_GWMH9P3.LCKFN.000_58_  Port=2
  RE_conf : Inport  Tag={'output',{'name','$I_RE_conf','class','ESR_VC/FCN_ARG','type','UInt8'},'date',737395.78910004627}  Description=_GWMH9P3.LCKFN.000_59_  Port=3
  RE_A0 : Inport  Tag={'output',{'name','$I_RE_A0','class','ESR_VC/FCN_ARG','type','Float32'},'date',737395.78706298606}  Description=_GWMH9P3.LCKFN.000_60_  Port=4
  Barr_range : Inport  Tag={'output',{'name','$I_Barr_range','class','ESR_VC/FCN_ARG','type','Float32'},'date',737395.79003777774}  Description=_GWMH9P3.LCKFN.000_61_  Port=5
  Barr_status : Inport  Tag={'output',{'name','$I_Barr_status','class','ESR_VC/FCN_ARG','type','UInt8'},'date',737395.79025012732}  Description=_GWMH9P3.LCKFN.000_62_  Port=6
  Barr_conf : Inport  Tag={'output',{'name','$I_Barr_conf','class','ESR_VC/FCN_ARG','type','UInt8'},'date',737395.79030952544}  Description=_GWMH9P3.LCKFN.000_63_  Port=7
  Barr_A0 : Inport  Tag={'output',{'name','$I_Barr_A0','class','ESR_VC/FCN_ARG','type','Float32'},'date',737395.79016039358}  Description=_GWMH9P3.LCKFN.000_64_  Port=8
  Gdr_range : Inport  Tag={'output',{'name','$I_Gdr_range','type','Float32'},'date',737395.79107519682}  Description=_GWMH9P3.LCKFN.000_65_  Port=9
  Gdr_status : Inport  Tag={'output',{'name','$I_Gdr_status','class','ESR_VC/FCN_ARG','type','UInt8'},'date',737395.79137348384}  Description=_GWMH9P3.LCKFN.000_66_  Port=10
  Gdr_conf : Inport  Tag={'output',{'name','$I_Gdr_conf','class','ESR_VC/FCN_ARG','type','UInt8'},'date',737395.7916990394}  Description=_GWMH9P3.LCKFN.000_67_  Port=11
  Gdr_A0 : Inport  Tag={'output',{'name','$I_Gdr_A0','class','ESR_VC/FCN_ARG','type','Float32'},'date',737395.7909677662}  Description=_GWMH9P3.LCKFN.000_68_  Port=12
  min_valid_range_m : Inport  Tag={'output',{'name','$I_min_valid_range_m','class','ESR_VC/FCN_ARG','type','UInt8'},'date',737395.78932809026}  Description=_GWMH9P3.LCKFN.000_69_  Port=13
  Max_Valid_Offset : Inport  Tag={'output',{'name','$I_Max_Valid_Offset','class','ESR_VC/FCN_ARG'},'date',737395.79202499997}  Description=_GWMH9P3.LCKFN.000_70_  Port=14
  Abs : Abs  Tag={'output',{'type','Float32'},'date',737394.50935303245}  Description=_GWMH9P3.LCKFN.000_71_
  Abs1 : Abs  Tag={'output',{'type','Float32'},'date',737394.50935375004}  Description=_GWMH9P3.LCKFN.000_72_
  Abs2 : Abs  Tag={'output',{'type','Float32'},'date',737394.50935401616}  Description=_GWMH9P3.LCKFN.000_73_
  Abs3 : Abs  Tag={'output',{'type','Float32'},'date',737394.5093542824}  Description=_GWMH9P3.LCKFN.000_74_
  Abs4 : Abs  Tag={'output',{'type','Float32'},'date',737394.50935456017}  Description=_GWMH9P3.LCKFN.000_75_
  Abs5 : Abs  Tag={'output',{'type','Float32'},'date',737394.5093551157}  Description=_GWMH9P3.LCKFN.000_76_
  Add1 : Sum  Tag={'output',{'type','UInt8'},'date',737395.47284584492}  Description=_GWMH9P3.LCKFN.000_77_  Inputs=+++
  Add3 : Sum  Tag={'output',{'type','Float32'},'date',737394.61890537036}  Description=_GWMH9P3.LCKFN.000_78_
  Add4 : Sum  Tag={'output',{'type','Float32'},'date',737394.61673247686}  Description=_GWMH9P3.LCKFN.000_79_
  Add5 : Sum  Tag={'output',{'type','Float32'},'date',737394.57922549767}  Description=_GWMH9P3.LCKFN.000_80_
  Gain : Gain  Tag={'output',{'type','UInt8'},'gain',{'type','Int32'},'date',737395.78289579856}  Description=_GWMH9P3.LCKFN.000_81_  Gain=4
  Gain1 : Gain  Tag={'output',{'type','UInt8'},'gain',{'type','Int32'},'date',737395.78314640047}  Description=_GWMH9P3.LCKFN.000_82_  Gain=2
  ME_LBARR_Chk : $bdroot/ME_Lane_Chk  SystemSampleTime=-1
  ME_LFGDR_Chk : $bdroot/ME_Lane_Chk  SystemSampleTime=-1
  ME_LRE_Chk : $bdroot/ME_Lane_Chk  SystemSampleTime=-1
  Relational Operator5 : RelationalOperator  Tag={'date',737393.51891306718}  Description=_GWMH9P3.LCKFN.000_83_  Operator=<  OutDataTypeStr=boolean  RndMeth=Nearest
  Relational Operator6 : RelationalOperator  Tag={'date',737393.51891327545}  Description=_GWMH9P3.LCKFN.000_84_  Operator=<  OutDataTypeStr=boolean  RndMeth=Nearest
  Relational Operator7 : RelationalOperator  Tag={'date',737393.518913507}  Description=_GWMH9P3.LCKFN.000_85_  Operator=<  OutDataTypeStr=boolean  RndMeth=Nearest
  Switch34 : Switch  Tag={'output',{'type','Float32'},'threshold',{'type','Int32'},'date',737395.47176994209}  Description=_GWMH9P3.LCKFN.000_86_  Criteria=u2 ~= 0
  Switch35 : Switch  Tag={'output',{'type','Float32'},'threshold',{'type','Int32'},'date',737395.47187481483}  Description=_GWMH9P3.LCKFN.000_87_  Criteria=u2 ~= 0
  Switch36 : Switch  Tag={'output',{'type','Float32'},'threshold',{'type','Int32'},'date',737395.47212880792}  Description=_GWMH9P3.LCKFN.000_88_  Criteria=u2 ~= 0
  Switch37 : Switch  Tag={'output',{'type','Float32'},'threshold',{'type','Int32'},'date',737395.4722498958}  Description=_GWMH9P3.LCKFN.000_89_  Criteria=u2 ~= 0
  Switch38 : Switch  Tag={'output',{'type','Float32'},'threshold',{'type','Int32'},'date',737395.47235892364}  Description=_GWMH9P3.LCKFN.000_90_  Criteria=u2 ~= 0
  Switch39 : Switch  Tag={'output',{'type','Float32'},'threshold',{'type','Int32'},'date',737395.47246385412}  Description=_GWMH9P3.LCKFN.000_91_  Criteria=u2 ~= 0
  k_SPP_clearance_FusGdr : Constant  Tag={'output',{'name','$P','class','EXTERN_CAL','type','Float32'},'date',737394.53117398149}  Description=_GWMH9P3.LCKFN.000_92_  Value=k_SPP_clearance_FusGdr  SampleTime=-1
  k_SPP_clearance_RE : Constant  Tag={'output',{'name','$P','class','EXTERN_CAL','type','Float32'},'date',737394.61885945604}  Description=_GWMH9P3.LCKFN.000_93_  Value=k_SPP_clearance_RE  SampleTime=-1
  k_SPP_clearance_VisBarr : Constant  Tag={'output',{'name','$P','class','EXTERN_CAL','type','Float32'},'date',737394.61815101851}  Description=_GWMH9P3.LCKFN.000_94_  Value=k_SPP_clearance_VisBarr  SampleTime=-1
  Min_offset_m : Outport  Tag={'output',{'name','$I_Min_offset_m','type','Float32'},'date',737395.79243659717}  Description=_GWMH9P3.LCKFN.000_95_
  Rdge_Barr_Sel : Outport  Tag={'output',{'name','$I_Rdge_Barr_Sel','type','UInt8'},'date',737395.79255524301}  Description=_GWMH9P3.LCKFN.000_96_  Port=2
  wires:
  ME_LRE_Chk/1 -> Switch34/2
  k_SPP_clearance_RE/1 -> Add3/1
  Add3/1 -> Switch34/1
  Add4/1 -> Switch35/1
  k_SPP_clearance_VisBarr/1 -> Add4/1
  ME_LBARR_Chk/1 -> Switch35/2
  Add5/1 -> Switch36/1
  ME_LFGDR_Chk/1 -> Switch36/2
  k_SPP_clearance_FusGdr/1 -> Add5/1
  Switch36/1 -> Abs2/1, Switch37/1
  Abs2/1 -> Relational Operator5/1
  Abs/1 -> Relational Operator5/2
  Relational Operator5/1 -> Switch37/2, Add1/3
  Abs3/1 -> Relational Operator6/1
  Abs1/1 -> Relational Operator6/2
  Relational Operator6/1 -> Switch38/2, Gain1/1
  Switch37/1 -> Switch38/3, Abs1/1
  Switch35/1 -> Abs3/1, Switch38/1
  Abs5/1 -> Relational Operator7/1
  Abs4/1 -> Relational Operator7/2
  Relational Operator7/1 -> Switch39/2, Gain/1
  Switch34/1 -> Abs5/1, Switch39/1
  Switch38/1 -> Switch39/3, Abs4/1
  Switch39/1 -> Min_offset_m/1
  min_valid_range_m/1 -> ME_LRE_Chk/4, ME_LBARR_Chk/4, ME_LFGDR_Chk/4
  Gain/1 -> Add1/1
  Gain1/1 -> Add1/2
  Add1/1 -> Rdge_Barr_Sel/1  "Rdge_Barr_Sel"
  RE_range/1 -> ME_LRE_Chk/1
  RE_staus/1 -> ME_LRE_Chk/2
  RE_conf/1 -> ME_LRE_Chk/3
  RE_A0/1 -> Add3/2
  Barr_A0/1 -> Add4/2
  Barr_range/1 -> ME_LBARR_Chk/1
  Barr_status/1 -> ME_LBARR_Chk/2
  Barr_conf/1 -> ME_LBARR_Chk/3
  Gdr_range/1 -> ME_LFGDR_Chk/1
  Gdr_status/1 -> ME_LFGDR_Chk/2
  Gdr_conf/1 -> ME_LFGDR_Chk/3
  Gdr_A0/1 -> Add5/2
  Max_Valid_Offset/1 -> [Max_Valid_Offset]
  [Max_Valid_Offset] -> Switch36/3, Switch37/3, Abs/1
  [Max_Valid_Offset] -> Switch35/3
  [Max_Valid_Offset] -> Switch34/3

== system LateralControl_fcns_lib/Signal_Sustain ==
  input : Inport  Description=_GWMAB30P4.LKAFN.000_316_
  sustain_time : Inport  Description=_GWMAB30P4.LKAFN.000_317_  Port=2
  Sustain_wo_reset : Stateflow chart  Description=_GWMAB30P4.LKAFN.000_319_  TreatAsAtomicUnit=on
  sustain_value : Outport  Description=_GWMAB30P4.LKAFN.000_323_
  wires:
  sustain_time/1 -> Sustain_wo_reset/2(sustain_time)
  Sustain_wo_reset/1(sustain_value) -> sustain_value/1
  input/1 -> Sustain_wo_reset/1(input)

== system LateralControl_fcns_lib/Signal_Sustain_With_Clear ==
  input : Inport  Description=_GWMAB30P4.LKAFN.000_295_
  sustain_time : Inport  Description=_GWMAB30P4.LKAFN.000_296_  Port=2
  clear : Inport  Description=_GWMAB30P4.LKAFN.000_297_  Port=3
  signal_sustain : Stateflow chart  Description=_GWMAB30P4.LKAFN.000_299_  TreatAsAtomicUnit=on
  sustain_value : Outport  Description=_GWMAB30P4.LKAFN.000_304_
  wires:
  clear/1 -> signal_sustain/3(clear)
  signal_sustain/1(sustain_value) -> sustain_value/1
  sustain_time/1 -> signal_sustain/2(sustain_time)
  input/1 -> signal_sustain/1(input)

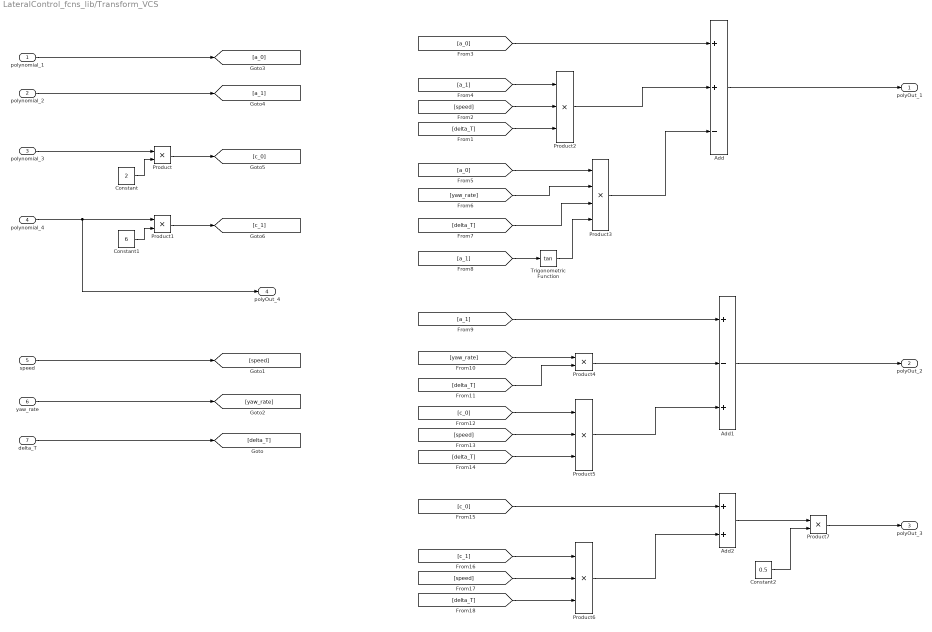
== system LateralControl_fcns_lib/Transform_VCS ==
  polynomial_1 : Inport  Description=_GWMH9P4.LCKFN.000_53_
  polynomial_2 : Inport  Description=_GWMH9P4.LCKFN.000_54_  Port=2
  polynomial_3 : Inport  Description=_GWMH9P4.LCKFN.000_55_  Port=3
  polynomial_4 : Inport  Description=_GWMH9P4.LCKFN.000_56_  Port=4
  speed : Inport  Description=_GWMH9P4.LCKFN.000_57_  Port=5
  yaw_rate : Inport  Description=_GWMH9P4.LCKFN.000_58_  Port=6
  delta_T : Inport  Description=_GWMH9P4.LCKFN.000_59_  Port=7
  Add : Sum  Tag={'output',{'type','Float32'},'date',737462.83802695607}  Description=_GWMH9P4.LCKFN.000_60_  Inputs=++-
  Add1 : Sum  Tag={'output',{'type','Float32'},'date',737462.83816357644}  Description=_GWMH9P4.LCKFN.000_61_  Inputs=+-+
  Add2 : Sum  Tag={'output',{'type','Float32'},'date',737462.83826973382}  Description=_GWMH9P4.LCKFN.000_62_
  Constant : Constant  Tag={'output',{'type','Int32'},'date',737462.49267282407}  Description=_GWMH9P4.LCKFN.000_63_  Value=2
  Constant1 : Constant  Tag={'output',{'type','Int32'},'date',737462.49267299764}  Description=_GWMH9P4.LCKFN.000_64_  Value=6
  Constant2 : Constant  Tag={'output',{'type','Int32'},'date',737462.49267318286}  Description=_GWMH9P4.LCKFN.000_65_  Value=0.5
  Product : Product  Tag={'output',{'type','Float32'},'date',737462.83772556717}  Description=_GWMH9P4.LCKFN.000_66_
  Product1 : Product  Tag={'output',{'type','Float32'},'date',737462.83779719903}  Description=_GWMH9P4.LCKFN.000_67_
  Product2 : Product  Tag={'output',{'type','Float32'},'date',737462.83785875002}  Description=_GWMH9P4.LCKFN.000_68_  Inputs=3
  Product3 : Product  Tag={'output',{'type','Float32'},'date',737462.83791134262}  Description=_GWMH9P4.LCKFN.000_69_  Inputs=4
  Product4 : Product  Tag={'output',{'type','Float32'},'date',737462.83807886578}  Description=_GWMH9P4.LCKFN.000_70_
  Product5 : Product  Tag={'output',{'type','Float32'},'date',737462.83812184026}  Description=_GWMH9P4.LCKFN.000_71_  Inputs=3
  Product6 : Product  Tag={'output',{'type','Float32'},'date',737462.8382226968}  Description=_GWMH9P4.LCKFN.000_72_  Inputs=3
  Product7 : Product  Tag={'output',{'type','Float32'},'date',737462.83833524305}  Description=_GWMH9P4.LCKFN.000_73_
  Trigonometric Function : Trigonometry  Tag={'output',{'type','Float32'},'date',737462.73073488427}  Description=_GWMH9P4.LCKFN.000_74_  Operator=tan
  polyOut_1 : Outport  Description=_GWMH9P4.LCKFN.000_75_
  polyOut_2 : Outport  Description=_GWMH9P4.LCKFN.000_76_  Port=2
  polyOut_3 : Outport  Description=_GWMH9P4.LCKFN.000_77_  Port=3
  polyOut_4 : Outport  Description=_GWMH9P4.LCKFN.000_78_  Port=4
  wires:
  polynomial_4/1 -> polyOut_4/1, Product1/1
  [speed] -> Product6/2
  Add/1 -> polyOut_1/1
  [delta_T] -> Product2/3
  speed/1 -> [speed]
  Product6/1 -> Add2/2
  Trigonometric Function/1 -> Product3/4
  Product4/1 -> Add1/2
  [delta_T] -> Product3/3
  [delta_T] -> Product5/3
  [c_1] -> Product6/1
  [speed] -> Product2/2
  Add1/1 -> polyOut_2/1
  Product1/1 -> [c_1]
  Product/1 -> [c_0]
  [yaw_rate] -> Product3/2
  Product5/1 -> Add1/3
  [a_1] -> Product2/1
  [speed] -> Product5/2
  delta_T/1 -> [delta_T]
  [c_0] -> Add2/1
  [c_0] -> Product5/1
  [delta_T] -> Product6/3
  Product2/1 -> Add/2
  Constant2/1 -> Product7/2
  Constant/1 -> Product/2
  polynomial_1/1 -> [a_0]
  polynomial_3/1 -> Product/1
  [a_0] -> Product3/1
  [a_0] -> Add/1
  [delta_T] -> Product4/2
  Product3/1 -> Add/3
  [a_1] -> Add1/1
  Constant1/1 -> Product1/2
  [yaw_rate] -> Product4/1
  Add2/1 -> Product7/1
  [a_1] -> Trigonometric Function/1
  yaw_rate/1 -> [yaw_rate]
  polynomial_2/1 -> [a_1]
  Product7/1 -> polyOut_3/1

== system LateralControl_fcns_lib/Trigger Hold Counter ==
  Trigger : Inport  Description=_GACA26P4.LCK.000_235_
  hold_time : Inport  Description=_GACA26P4.LCK.000_236_  Port=2
  Trigger Hold : Stateflow chart  TreatAsAtomicUnit=on
  Out : Outport  Description=_GACA26P4.LCK.000_241_
  Counter : Outport  Description=_GACA26P4.LCK.000_242_  Port=2
  wires:
  Trigger Hold/1(Out) -> Out/1
  hold_time/1 -> Trigger Hold/2(hold_time)
  Trigger Hold/2(count) -> Counter/1
  Trigger/1 -> Trigger Hold/1(Trigger)

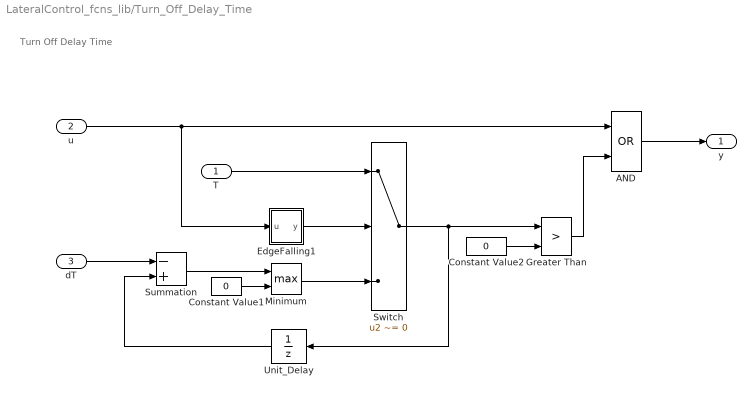
== system LateralControl_fcns_lib/Turn_Off_Delay_Time ==
  note: Turn Off Delay Time
  T : Inport
  u : Inport  Port=2
  dT : Inport  Port=3
  AND : Logic  Operator=OR  OutDataTypeStr=boolean
  Constant Value1 : Constant  Value=0  OutDataTypeStr=Inherit: Inherit via back propagation
  Constant Value2 : Constant  Value=0  OutDataTypeStr=Inherit: Inherit via back propagation
  EdgeFalling1 : Subsystem  mask(EdgeFalling){vinit=0}
      mask prompts: vinit "Init Codition"
      mask help: The output indicates true if the logical input value changes from true to false. Input1=Value (u).
      settings: AttributesFormatString=<Init Codition = %<vinit>>  RTWSystemCode=Inline
      mask Help: web(char(which([char(get_param(gcb,'MaskType')),'.html'])));
      mask Display:
      | color('blue');
      | plot([0.15 0.5 0.5 0.85], [0.9 0.9 0.15 0.15])
      | plot([0.38 0.5 0.62], [0.65 0.4 0.65])
  Greater Than : RelationalOperator  Operator=>  OutDataTypeStr=boolean  RndMeth=Nearest  InputSameDT=on
  Minimum : MinMax  Function=max  Inputs=2  RndMeth=Zero  SaturateOnIntegerOverflow=on  InputSameDT=on
  Summation : Sum  Inputs=-+  RndMeth=Zero  SaturateOnIntegerOverflow=on  InputSameDT=on  OutDataTypeStr=Inherit: Same as first input
  Switch : Switch  Criteria=u2 ~= 0  Threshold=1  RndMeth=Zero  InputSameDT=on
      settings: AttributesFormatString=<%<Criteria>>
  Unit_Delay : UnitDelay  SampleTime=-1
      settings: AttributesFormatString=|
      | <init value = %<InitialCondition>>
      | <sample time = %<SampleTime>>
  y : Outport
  wires:
  Minimum/1 -> Switch/3
  dT/1 -> Summation/1
  Switch/1 -> Unit_Delay/1, Greater Than/1
  Greater Than/1 -> AND/2
  AND/1 -> y/1
  u/1 -> EdgeFalling1/1(u), AND/1
  Unit_Delay/1 -> Summation/2
  Constant Value2/1 -> Greater Than/2
  Summation/1 -> Minimum/1
  Constant Value1/1 -> Minimum/2
  EdgeFalling1/1(y) -> Switch/2
  T/1 -> Switch/1
